simulink model "trial3"  (R2020a)
settings: Solver=VariableStepAuto  StartTime=0.0  StopTime=10.0  RelTol=1e-3
undefined symbols (not defined in the file): A, F, T
settings Model: Creator="mukesh  thota"  LastModifiedBy="mukesh  thota"

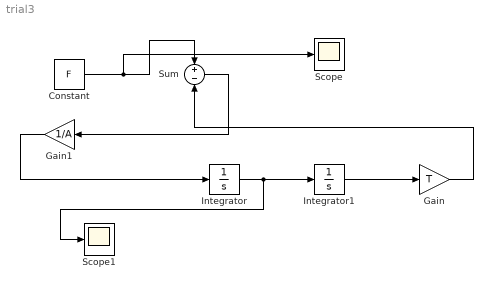
== system trial3 ==
  Constant : Constant  Value=F
  Gain : Gain  Gain=T
  Gain1 : Gain  Gain=1/A
  Integrator : Integrator
  Integrator1 : Integrator
  Scope : Scope
  Scope1 : Scope
  Sum : Sum  Inputs=+-
  wires:
  Gain1/1 -> Integrator/1
  Integrator/1 -> Scope1/1, Integrator1/1
  Integrator1/1 -> Gain/1
  Gain/1 -> Sum/2
  Constant/1 -> Scope/1, Sum/1
  Sum/1 -> Gain1/1
